simulink model "integrator_ex"  (R2022b)
settings: Solver=VariableStepAuto  StartTime=0.0  StopTime=10.0  MaxStep=.01  RelTol=1e-3
settings Model: Creator=Brigosha_Guest  LastModifiedBy=Brigosha_Guest

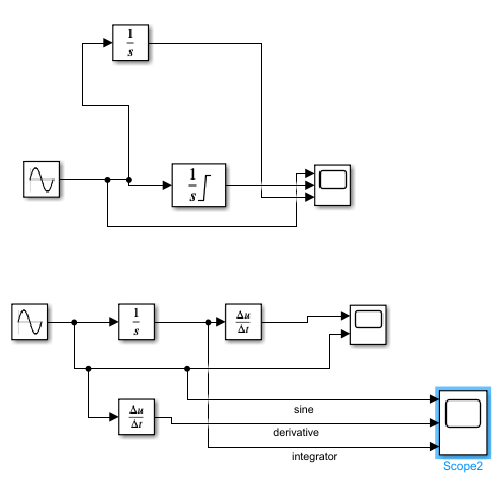
[thumbnail: Simulink's stored preview of the top-level diagram]
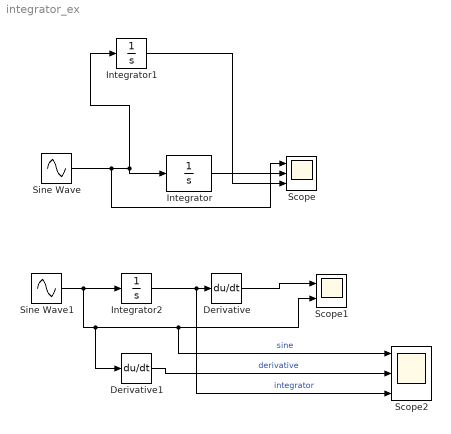
== system integrator_ex ==
  Derivative : Derivative
  Derivative1 : Derivative
  Integrator : Integrator  LimitOutput=on  UpperSaturationLimit=1  LowerSaturationLimit=-1
  Integrator1 : Integrator  UpperSaturationLimit=1  LowerSaturationLimit=-1
  Integrator2 : Integrator  UpperSaturationLimit=1  LowerSaturationLimit=-1
  Scope : Scope  NumInputPorts=3
  Scope1 : Scope  NumInputPorts=2
  Scope2 : Scope  NumInputPorts=3
  Sine Wave : Sin  SampleTime=0
  Sine Wave1 : Sin  SampleTime=0
  wires:
  Sine Wave/1 -> Scope/1, Integrator1/1, Integrator/1
  Integrator/1 -> Scope/2
  Integrator1/1 -> Scope/3
  Sine Wave1/1 -> Derivative1/1, Scope2/1, Scope1/2, Integrator2/1  "sine"
  Integrator2/1 -> Scope2/3, Derivative/1  "integrator"
  Derivative/1 -> Scope1/1
  Derivative1/1 -> Scope2/2  "derivative"
